simulink model "LQR_and_Trcking_control"  (R2023b)
settings: Solver=VariableStepAuto  StartTime=0.0  StopTime=100.0  RelTol=1e-3
values from neighbouring files (symbols this model uses):
  A = double(A)    [consistent.m]    (also in dyn_model_mark.m)
  B = double(B)    [consistent.m]    (also in dyn_model_mark.m)
  x1_bar = 0    [consistent.m]    (also in dyn_model_mark.m)
  x3_bar = 0    [consistent.m]    (also in dyn_model_mark.m = 3.14159265359)
undefined symbols (not defined in the file or in its folder): A_uns, B_uns, K_lq_track, K_lq_track_uns, K_lq_uns, x1_bar_uns, x3_bar_uns
libraries: simulink_extras x9, simulink x1
settings Model: Creator=Mark  LastModifiedBy=Mark

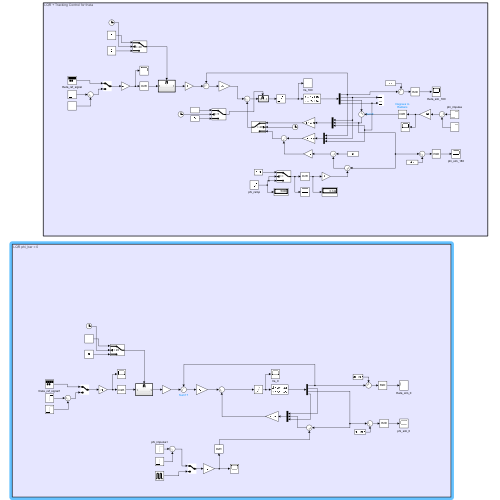
[thumbnail: Simulink's stored preview of the top-level diagram]
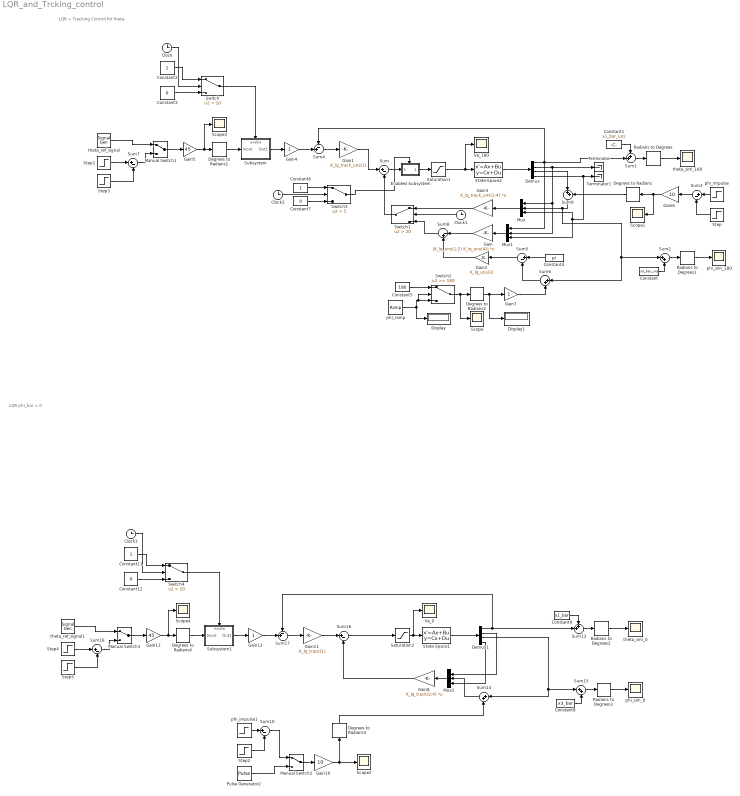
== system LQR_and_Trcking_control ==
  note: LQR + Tracking Control for theta
  note: LQR phi_bar = 0
  Clock{,1..3} (4 alike) : Clock
  Constant : Constant  Value=x3_bar_uns
  Constant1 : Constant  Value=x1_bar_uns
  Constant11 : Constant
  Constant12 : Constant  Value=0
  Constant2 : Constant
  Constant3 : Constant  Value=0
  Constant4 : Constant  Value=pi
  Constant5 : Constant  Value=180
  Constant6 : Constant
  Constant7 : Constant  Value=0
  Constant8 : Constant  Value=x3_bar
  Constant9 : Constant  Value=x1_bar
  Degrees to Radians{,1..4} (5 alike) : simulink_extras/Transformations/Degrees to Radians
  Demux : Demux
  Demux1 : Demux
  Display : Display
  Display1 : Display
  Enabled Subsystem : Subsystem  TreatAsAtomicUnit=on
  Gain : Gain  Gain=[K_lq_uns(1:2) K_lq_uns(4)]  Multiplication=Matrix(K*u) (u vector)
  Gain1 : Gain  Gain=K_lq_track_uns(1)
  Gain10 : Gain  Gain=10
  Gain11 : Gain  Gain=K_lq_track(1)
  Gain12 : Gain
  Gain13 : Gain  Gain=45
  Gain2 : Gain  Gain=K_lq_uns(3)
  Gain3 : Gain  Gain=K_lq_track_uns(2:4)  Multiplication=Matrix(K*u) (u vector)
  Gain4 : Gain
  Gain5 : Gain  Gain=45
  Gain6 : Gain  Gain=10
  Gain7 : Gain
  Gain8 : Gain  Gain=K_lq_track(2:4)  Multiplication=Matrix(K*u) (u vector)
  Manual Switch1 : ManualSwitch
  Manual Switch2 : ManualSwitch
  Manual Switch3 : ManualSwitch
  Mux : Mux  Inputs=3
  Mux1 : Mux  Inputs=3
  Mux2 : Mux  Inputs=3
  Pulse Generator2 : DiscretePulseGenerator  PulseType=Time based  Period=4  PulseWidth=50  PhaseDelay=10
  Radians to Degrees{,1..3} (4 alike) : simulink_extras/Transformations/Radians to Degrees
  Saturation1 : Saturate  UpperLimit=10  LowerLimit=-10
  Saturation2 : Saturate  UpperLimit=10  LowerLimit=-10
  Scope{,1..4} (5 alike) : Scope
  State-Space1 : StateSpace  A=A  B=B  C=eye(4)  D=zeros(4,1)  InitialCondition=[0 0 0 0]
  State-Space2 : StateSpace  A=A_uns  B=B_uns  C=eye(4)  D=zeros(4,1)  InitialCondition=[0 0 0 0]
  Step : Step  Time=30.05  SampleTime=0
  Step1 : Step  Time=20  SampleTime=0
  Step2 : Step  Time=30.5  SampleTime=0
  Step3 : Step  Time=50  After=0  SampleTime=0
  Step4 : Step  Time=20  SampleTime=0
  Step5 : Step  Time=50  After=0  SampleTime=0
  Subsystem : Subsystem
  Subsystem1 : Subsystem
  Sum{,3,5,7,10,16,18} (7 alike) : Sum  Inputs=|+-
  Sum1 : Sum  Inputs=++|
  Sum13 : Sum  Inputs=++|
  Sum{2,6,9,14..15} (5 alike) : Sum  Inputs=|++
  Sum17 : Sum  Inputs=-+|
  Sum4 : Sum  Inputs=-+|
  Sum8 : Sum  Inputs=|-+
  Switch : Switch  Criteria=u2 > Threshold  Threshold=20  SaturateOnIntegerOverflow=off  InputSameDT=off
  Switch1 : Switch  Criteria=u2 > Threshold  Threshold=20  SaturateOnIntegerOverflow=off  InputSameDT=off
  Switch2 : Switch  Threshold=180  SaturateOnIntegerOverflow=off  InputSameDT=off
  Switch3 : Switch  Criteria=u2 > Threshold  Threshold=5  SaturateOnIntegerOverflow=off  InputSameDT=off
  Switch4 : Switch  Criteria=u2 > Threshold  Threshold=20  SaturateOnIntegerOverflow=off  InputSameDT=off
  Terminator : Terminator
  Terminator1 : Terminator
  Va_0 : Scope
  Va_180 : Scope
  phi_impulse : Step  Time=30  SampleTime=0
  phi_impulse1 : Step  Time=30  SampleTime=0
  phi_ramp : simulink/Sources/Ramp  slope=50  start=0  InitialOutput=0
  phi_sim_0 : Scope
  phi_sim_180 : Scope
  theta_ref_signal : SignalGenerator  Frequency=0.1
  theta_ref_signal1 : SignalGenerator  Frequency=0.1
  theta_sim_0 : Scope
  theta_sim_180 : Scope
  wires:
  Degrees to Radians/1 -> Sum9/2
  Constant/1 -> Sum2/2
  Sum1/1 -> Radians to Degrees/1
  Radians to Degrees1/1 -> phi_sim_180/1
  Saturation1/1 -> State-Space2/1, Va_180/1
  Demux/1 -> Mux1/1, Sum1/2, Sum4/1
  Constant1/1 -> Sum1/1
  Sum2/1 -> Radians to Degrees1/1
  Switch1/1 -> Sum/2
  Enabled Subsystem/1(Out1) -> Saturation1/1
  Gain6/1 -> Scope1/1, Degrees to Radians/1
  State-Space2/1 -> Demux/1
  Radians to Degrees/1 -> theta_sim_180/1
  Sum3/1 -> Gain6/1
  Sum/1 -> Enabled Subsystem/1(In1)
  Step/1 -> Sum3/2
  phi_impulse/1 -> Sum3/1
  Demux/2 -> Terminator/1, Mux1/2, Mux/1
  Demux/4 -> Mux1/3, Mux/3, Terminator1/1
  Switch/1 -> Subsystem/Enable
  Constant2/1 -> Switch/1
  Constant3/1 -> Switch/3
  Clock/1 -> Switch/2
  Clock1/1 -> Switch1/2
  Gain3/1 -> Switch1/1
  Sum4/1 -> Gain1/1
  Gain1/1 -> Sum/1
  Subsystem/1(Out1) -> Gain4/1
  Mux/1 -> Gain3/1
  Gain4/1 -> Sum4/2
  theta_ref_signal/1 -> Manual Switch1/1
  Step3/1 -> Sum7/2
  Manual Switch1/1 -> Gain5/1
  Step1/1 -> Sum7/1
  Sum7/1 -> Manual Switch1/2
  Gain5/1 -> Scope3/1, Degrees to Radians1/1
  Degrees to Radians1/1 -> Subsystem/1(Input)
  Constant5/1 -> Switch2/1
  Degrees to Radians2/1 -> Gain7/1, Display1/1
  Switch2/1 -> Scope/1, Degrees to Radians2/1
  phi_ramp/1 -> Display/1, Switch2/2, Switch2/3
  Sum9/1 -> Mux/2, Sum2/1, Sum6/1
  Constant4/1 -> Sum5/1
  Mux1/1 -> Gain/1
  Gain7/1 -> Sum6/2
  Gain/1 -> Sum8/1
  Constant6/1 -> Switch3/1
  Constant7/1 -> Switch3/3
  Switch3/1 -> Enabled Subsystem/Enable
  Clock2/1 -> Switch3/2
  Sum6/1 -> Sum5/2
  Sum5/1 -> Gain2/1
  Sum8/1 -> Switch1/3
  Gain2/1 -> Sum8/2
  Demux/3 -> Sum9/1
  Mux2/1 -> Gain8/1
  Constant8/1 -> Sum15/2
  Sum10/1 -> Manual Switch2/1
  Radians to Degrees3/1 -> phi_sim_0/1
  phi_impulse1/1 -> Sum10/1
  Sum15/1 -> Radians to Degrees3/1
  Gain10/1 -> Scope2/1, Degrees to Radians3/1
  Step2/1 -> Sum10/2
  Pulse Generator2/1 -> Manual Switch2/2
  Demux1/2 -> Mux2/1
  Saturation2/1 -> Va_0/1, State-Space1/1
  Radians to Degrees2/1 -> theta_sim_0/1
  Demux1/4 -> Mux2/3
  Degrees to Radians3/1 -> Sum14/2
  Demux1/1 -> Sum13/2, Sum17/1
  Constant9/1 -> Sum13/1
  State-Space1/1 -> Demux1/1
  Demux1/3 -> Sum14/1, Sum15/1
  Sum16/1 -> Saturation2/1
  Sum13/1 -> Radians to Degrees2/1
  Sum14/1 -> Mux2/2
  Manual Switch2/1 -> Gain10/1
  Gain8/1 -> Sum16/2
  Sum18/1 -> Manual Switch3/2
  Step4/1 -> Sum18/1
  Constant12/1 -> Switch4/3
  Gain13/1 -> Scope4/1, Degrees to Radians4/1
  Clock3/1 -> Switch4/2
  Switch4/1 -> Subsystem1/Enable
  Sum17/1 -> Gain11/1
  Degrees to Radians4/1 -> Subsystem1/1(Input)
  Manual Switch3/1 -> Gain13/1
  Gain12/1 -> Sum17/2
  theta_ref_signal1/1 -> Manual Switch3/1
  Gain11/1 -> Sum16/1
  Constant11/1 -> Switch4/1
  Step5/1 -> Sum18/2
  Subsystem1/1(Out1) -> Gain12/1

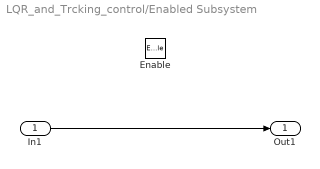
== system LQR_and_Trcking_control/Enabled Subsystem ==
  In1 : Inport
  Enable : EnablePort
  Out1 : Outport
  wires:
  In1/1 -> Out1/1

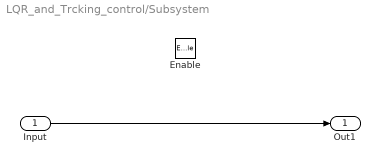
== system LQR_and_Trcking_control/Subsystem ==
  Input : Inport
  Enable : EnablePort
  Out1 : Outport
  wires:
  Input/1 -> Out1/1

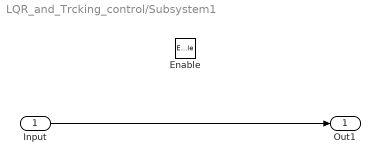
== system LQR_and_Trcking_control/Subsystem1 ==
  Input : Inport
  Enable : EnablePort
  Out1 : Outport
  wires:
  Input/1 -> Out1/1
